simulink model "mOvertakeManeuver"  (R2018b)
settings: Solver=VariableStepAuto  StartTime=0.0  StopTime=simTime  RelTol=1e-3
PreLoadFcn:
  | load 'tableStructure.mat'
InitFcn:
  | modelParams
  | clear markedSmartActorCount;
values from neighbouring files (symbols this model uses):
  initYPos = (scene.RoadNetwork.RoadCenters(1, 2) - laneWidth / 2)    [modelParams.m]
  initYPosRogue = (scene.RoadNetwork.RoadCenters(1, 2) - laneWidth / 2)    [modelParams.m]
  laneWidth = roadWidth / (scene.RoadNetwork.NumMarkings - 1)    [modelParams.m]
  maxLanes = 10    [modelParams.m]
  maxVehicles = 25    [modelParams.m]
  minOvertakeProximity = 50    [modelParams.m]
  numActors = length(scene.vehiclePoses(1).ActorPoses)    [modelParams.m]    (also in sessionLogReader.m = numel(inStruct); visualizer.m = numel(actors))
  numAddedRogueActors = 0    [modelParams.m]
  numLanes = scene.RoadNetwork.NumLanes    [modelParams.m]    (also in sessionLogReader.m = numMarkings-1)
  numSmartActors = 0    [modelParams.m]
  numSmartActorsDM = 0    [modelParams.m]
  rogueActorIdBase = 4000    [modelParams.m]
  safeTimeGap = 1.4    [modelParams.m]
  sensorRange = 600    [modelParams.m]
  smartActors = 0    [modelParams.m]    (also in sessionLogReader.m = repmat(actorPoses(1), [obj.NumSmartActors, 1]))
  smartActorsDM = 0    [modelParams.m]    (also in sessionLogReader.m = repmat(actorPoses(1), [obj.NumSmartActorsDM, 1]))
  standStillGap = 10    [modelParams.m]
  W_SPEC = [Ln1;vdes;vmax;AXadd;AXmult;BXadd;BXmult;EXadd;EXmult;CXconst;CXadd;CXmult;OPDVmult;OPDVadd;BNULLmult;BMAXmult;FAKTORVmult;BMINadd;BMINmult;      RND1n;RND2n;RND3n;RND4n;NRND]    [wiedemannParams.m]
undefined symbols (not defined in the file or in its folder): actorPoseInit, addedRogueVelocity, addedRogueXPosition, DiscIntNeverNeededParam
libraries: dataTableBlockslib x2, mpcadaslib x1
(part 3 of 3)

== stateflow chart mOvertakeManeuver/Smart Actor/Smart Actor system/Planner/Plan Library and its evaluation/Plan 1/Plan 1: Overtake Maneuver ==
  settings: executeAtInitialization=1
  state Overtake maneuver plan: [group]
    This plan is a sequential execution of 3 sub-plans (once overtake feasibility check is positive):
    (i) Merging into opposite direction lane.
    (ii) Accelerate on oppposite direction lane to accumulate sufficient gap with respect to vehicle it is going to overtake by moving parallel to it.
    (iii) Merge back into the correct lane.
    executionFlag = 1 indicates that plan has to be executed
    executionFlag = 0 indicates that only entry condition has to be tested
    checkOvertakeFeasibility : This function checks whether it is possible for the the smart car to overtake at this moment based on the current environment.
  state [feasibilityFlag,timeOppLane] = checkOvertakeFeasibility(currPose) [function]
  state FeasibilityCheckofOvertakeManuver
    entry:
    conditionCheck = 0;
    timeOppLane = 0; % Time during which smart car move on left lane
    % (opposite direction lane) for overtaking.
    during:
    [conditionCheck, timeOppLane] = checkOvertakeFeasibility(currPose);
  state MergeCorrectLane
    %Merge back into correct lane
    entry:
    rightLaneCenterY = getRightLane(currPose);
    overtakeCompleted = 0;
    commandAngle = -45;
    accel = 0;
    during:
    % Smart vehicle reached the correct lane
    if(currPose.Position(2) <= rightLaneCenterY)
    commandAngle = 0;
    % This marks completion of overtake maneuver.
    overtakeCompleted = 1;
    end
    exit:
    planStatus = 0;
  state MergeOppLane
    % Merge into opposite direction
    % lane for initiating overtake
    entry:
    leftLaneCenterY = getLeftLane(currPose);
    mergeCompleted = 0;
    ACCTrigger = 0;
    planStatus = 1;
    % Move towards adjacen lane at 45 degrees.
    commandAngle = 45;
    accel = 0;
    during:
    if( currPose.Position(2) >= leftLaneCenterY)
    mergeCompleted = 1;
    end
  state AccelerateOnOppLane
    % Accelerate on opposite direction lane to overtake the
    % chosen rogue vehicle by moving parallel to it
    entry:
    accel = maxAcceleration;
    commandAngle = 0;
    oppLaneMovementCompleted = 0;
    during:
    % If  smart vehicle reached maximum Velocity
    if currPose.Velocity(1) >= maxVelocity
    %set acceleration to zero
    accel = 0;
    end
  (default) -> FeasibilityCheckofOvertakeManuver
  MergeCorrectLane -> FeasibilityCheckofOvertakeManuver : [overtakeCompleted==1]
  FeasibilityCheckofOvertakeManuver -> MergeOppLane : [conditionCheck == 1 && executionFlag == 1] % Start overtaking as feasibilty check is successful
  AccelerateOnOppLane -> MergeCorrectLane : [after(timeOppLane,sec)]
  MergeOppLane -> AccelerateOnOppLane : [mergeCompleted== 1]
  data: feasibilityFlag function_output; currPose function_input Bus: Vehicle size=1; timeOppLane function_output; executionFlag input; accel output; conditionCheck output; commandAngle output; maxAcceleration parameter; oppLaneMovementCompleted local; overtakeCompleted local; maxVelocity parameter; planStatus output; ACCTrigger output; currPose input Bus: Vehicle; leftLaneCenterY local; mergeCompleted local; rightLaneCenterY local; timeOppLane local

== matlab function mOvertakeManeuver/Scene Management/Publish To Data Table/Write inital pose from session-logs into data-table ==
  data: actorPoseInit parameter Bus: Vehicle; numActors parameter; addedRogueXPosition parameter; addedRogueVelocity parameter; initYPosRogue parameter; numAddedRogueActors parameter; rogueActorIdBase parameter
function initializePoseDataTable(actorPoseInit, numActors, addedRogueXPosition, addedRogueVelocity, initYPosRogue, numAddedRogueActors, rogueActorIdBase)
% Write initial poses of the actors in the data-table

% actorPoseInit - Initial pose information of driving session-log actors.
% numActors - Total actors in driving scenario session log.
persistent init;
if(isempty(init))
    init = false;
    % Write initial poses of session log actors into the data-table. 
    for k = 1 : numActors
        setActorTableEntry(actorPoseInit(k).ActorID,actorPoseInit(k));
    end
    
    % Write initial poses of added rogue actors into the data-table.
    actorInfo = struct('ActorID', 0, 'Position', [0 0 0], ...
        'Velocity', [0 0 0], 'Roll', 0, 'Pitch', 0, 'Yaw', 0, ...
        'AngularVelocity', [0 0 0]);
    for i = 1 : numAddedRogueActors
        actorInfo.ActorID = rogueActorIdBase + i;
        actorInfo.Position = [addedRogueXPosition(i) initYPosRogue 0];
        actorInfo.Velocity = [addedRogueVelocity(i) 0 0];
        setActorTableEntry(actorInfo.ActorID, actorInfo);
    end
end

== stateflow chart mOvertakeManeuver/Smart Actor/Smart Actor system/Planner/Plan Library and its evaluation/Plan 2/Plan 2: Movement on correct lane ==
  settings: executeAtInitialization=1
  state Plan to continue the movement on the correct lane. [group]
    - If there is no vehicle ahead, move at max acceleration to reach max velocity
    - Otherwise, set AdaptiveCruiseControl trigger flag so that acceleration is governed by ACC
    block to follow the vehicle ahead while keeping safe gap.
  (default) -> (junction 159)
  (junction 159) -> (junction 150) [order 1] : [executionFlag == 1]  % Whether to execute plan
  (junction 159) -> (junction 152) [order 2] : {
      |     conditionCheck = 1; % Default plan hence no condition check.
      | }
  (junction 150) -> (junction 186) : {
      |       accel = 0;
      |       commandAngle = 0;
      |       % Get vehicles ahead
      |       [numVeh vehiclesAheadInfo] = getVehAheadSameLaneSorted(currPose);
      |       i=1;
      | }
  (junction 186) -> (junction 187) [order 1] : [i<=numVeh]
  (junction 189) -> (junction 186) : {
      |      i=i+1;
      | }
  (junction 186) -> (junction 154) [order 2]
  (junction 187) -> (junction 189) : {
      |     % Convert to self-centered pose
      |      vehiclesAheadInfo(i) = ...
      |      globalToSelfCentered(currPose, vehiclesAheadInfo(i));
      | }
  (junction 154) -> (junction 155) [order 1] : [numVeh == 0 ] % If no vehicle ahead
  (junction 154) -> (junction 181) [order 2] : {
      |   % Set ACC trigger so that controller invokes ACC
      |   % to get desired acceleration for safe gap
      |   ACCTrigger = 1;
      | }
  (junction 155) -> (junction 157) : {
      | accel = maxAcceleration;
      | ACCTrigger = 0;
      | }
  (junction 157) -> (junction 173) [order 1] : [currPose.Velocity(1) >= maxVelocity]
      |        % If crossed max velocity
  (junction 157) -> (junction 170) [order 2]
  (junction 173) -> (junction 163) : {
      |  accel = 0;
      | }
  (junction 152) -> (junction 153) [order 1] : [conditionCheck == 1]
  (junction 152) -> (junction 178) [order 2]
  (junction 153) -> (junction 156) : {
      |    accel = 0;
      |    commandAngle = 0;
      | }
  (junction 170) -> (junction 181)
  (junction 163) -> (junction 170)
  (junction 181) -> (junction 184) : {
      |      planStatus = 0;
      | }
  (junction 156) -> (junction 178)
  (junction 184) -> (junction 156)
  data: executionFlag input; accel output; conditionCheck output; commandAngle output; maxAcceleration parameter; maxVelocity parameter; planStatus output; ACCTrigger output; currPose input Bus: Vehicle; vehiclesAheadInfo local Bus: Vehicle; numVeh local; i local

== matlab function mOvertakeManeuver/Smart Actor/Smart Actor system/Planner/Plan selector/Choose plan ==
  data: planId output; currPose input; numPlans parameter
function planId = findFeasiblePlan(currPose, numPlans)
% Find a plan which has highest priority and is feasible based on entry
% condition
planId = 0;
executionFlag = 0; % Only feasibility of plan is checked, plan is not executed

% Loop through all the plans in priority order, to select one
for index = 1 : numPlans
    [~, planCheck, ~, ~] = evaluatePlan(index, executionFlag, currPose);
    if(planCheck == 1)
        planId = index;
        return;
    end
end

== matlab function mOvertakeManeuver/Smart Actor/Load Initial Pose ==
  data: initPose output Bus: Vehicle; smartActorId parameter; actorPoseInit parameter; initYPos parameter
function initPose = loadInitPose(smartActorId, actorPoseInit, initYPos)
% Write initial pose entry into the actor pose table and return the same

persistent pose;
if(isempty(pose))
    % Read the initial pose info
    pose = struct('ActorID', smartActorId, 'Position', [actorPoseInit(smartActorId).Position(1) initYPos actorPoseInit(smartActorId).Position(3)], ...
        'Velocity', abs(actorPoseInit(smartActorId).Velocity), 'Roll', ...
        actorPoseInit(smartActorId).Roll, 'Pitch', actorPoseInit(smartActorId).Pitch, ...
        'Yaw', 0, 'AngularVelocity', actorPoseInit(smartActorId).AngularVelocity);
    setActorTableEntry(smartActorId, pose);
end
initPose = pose;
end

== matlab function mOvertakeManeuver/Smart Actor/Write pose to Data-Table ==
  data: pose input Bus: Vehicle
function publishUpdatedPose(pose)
% Update the actor pose in the data-table
setActorTableEntry(pose.ActorID, pose);
end
